simulink model "Observer"  (R2018b)
settings: Solver=VariableStepAuto  StartTime=0.0  StopTime=10.0  RelTol=1e-3
values from neighbouring files (symbols this model uses):
  A3 = [0  1  0; 0  0  1; 4374  -81  -36]    [A01633926.mat]    (also in TodoJunto.mat; final2 FUNCIONA.mat)
  B3 = [0 0 1]    [A01633926.mat]    (also in TodoJunto.mat; final2 FUNCIONA.mat)
  C3 = [39.6 4 0]    [A01633926.mat]    (also in TodoJunto.mat; final2 FUNCIONA.mat)
  K3 = [4380 -70 -30]    [A01633926.mat]    (also in TodoJunto.mat; final2 FUNCIONA.mat)
  L3 = [0.25002206018 -3.22521839578 129.179662118]    [TodoJunto.mat]    (also in final2 FUNCIONA.mat)
libraries: cstblocks x1
settings Model: Creator=Abraham Pérez  LastModifiedBy=Abraham Pérez

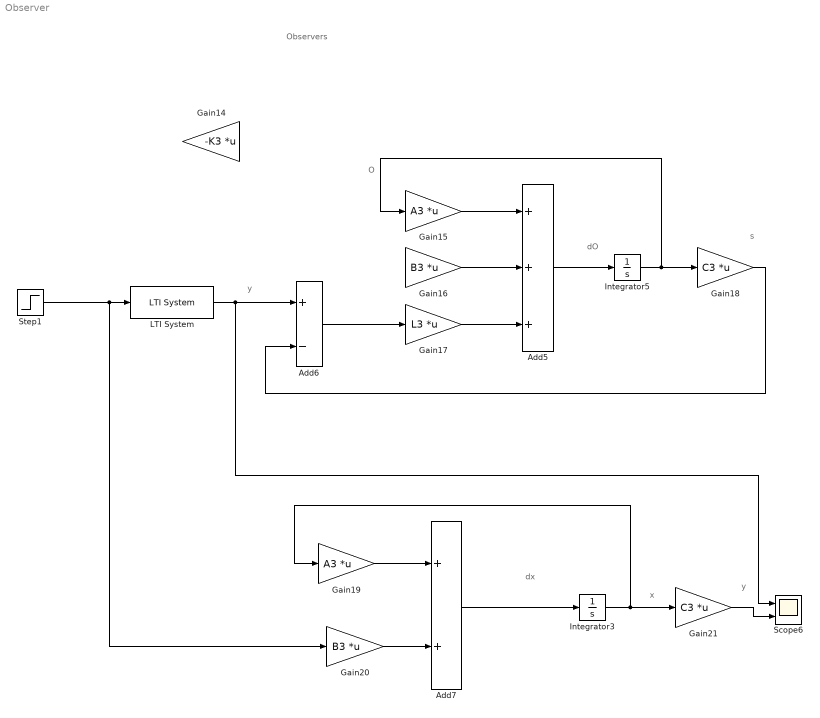
== system Observer ==
  note: y
  note: dO
  note: s
  note: O
  note: y
  note: dx
  note: x
  note: Observers
  Add5 : Sum  Inputs=+++
  Add6 : Sum  Inputs=+-
  Add7 : Sum
  Gain14 : Gain  Gain=-K3  Multiplication=Matrix(K*u)
  Gain15 : Gain  Gain=A3  Multiplication=Matrix(K*u)
  Gain16 : Gain  Gain=B3  Multiplication=Matrix(K*u)
  Gain17 : Gain  Gain=L3  Multiplication=Matrix(K*u)
  Gain18 : Gain  Gain=C3  Multiplication=Matrix(K*u)
  Gain19 : Gain  Gain=A3  Multiplication=Matrix(K*u)
  Gain20 : Gain  Gain=B3  Multiplication=Matrix(K*u)
  Gain21 : Gain  Gain=C3  Multiplication=Matrix(K*u)
  Integrator3 : Integrator
  Integrator5 : Integrator
  LTI System : cstblocks/LTI System  sys=G3  IC=[]
  Scope6 : Scope  NumInputPorts=2
  Step1 : Step  After=0  SampleTime=0
  wires:
  Integrator5/1 -> Gain18/1, Gain15/1
  Gain15/1 -> Add5/1
  Gain20/1 -> Add7/2
  Add6/1 -> Gain17/1
  Gain18/1 -> Add6/2
  LTI System/1 -> Scope6/1, Add6/1
  Gain17/1 -> Add5/3
  Add7/1 -> Integrator3/1
  Integrator3/1 -> Gain19/1, Gain21/1
  Gain16/1 -> Add5/2
  Step1/1 -> Gain20/1, LTI System/1
  Add5/1 -> Integrator5/1
  Gain21/1 -> Scope6/2
  Gain19/1 -> Add7/1
